simulink subsystem "StateSpaceControllerNominal_SubSystem"  (R2020b)
settings: Solver=VariableStepAuto  StartTime=0.0  StopTime=10.0  RelTol=1e-3
values from neighbouring files (symbols this model uses):
  K = place(A,B,p)    [StateSpaceControllerNominalCont.m]    (also in StateSpaceControllerNominalDigital.m; StateSpaceControllerNominalDirectDigital.m = place(Phi,Gamma,p); StateSpaceControllerRobustCont.m; StateSpaceControllerRobustDigital.m)
  Nu = reshape(Nu,[],1)    [StateSpaceControllerNominalCont.m]    (also in StateSpaceControllerNominalDigital.m; StateSpaceControllerNominalDirectDigital.m; StateSpaceControllerRobustCont.m; StateSpaceControllerRobustDigital.m)
  Nx = reshape(Nx,[],1)    [StateSpaceControllerNominalCont.m]    (also in StateSpaceControllerNominalDigital.m; StateSpaceControllerNominalDirectDigital.m; StateSpaceControllerRobustCont.m; StateSpaceControllerRobustDigital.m)
undefined symbols (not defined in the file or in its folder): rpm2rads
settings Model: Creator=umberto  LastModifiedBy=umberto

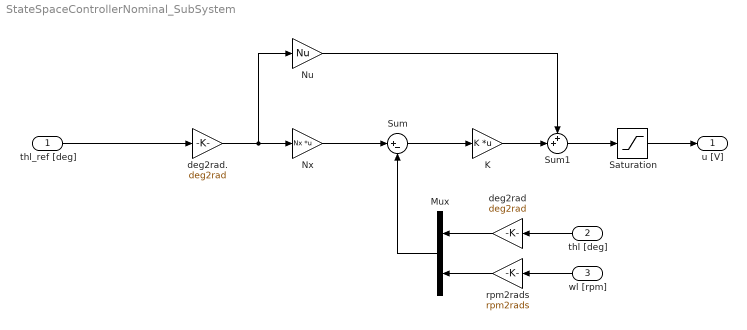
== system StateSpaceControllerNominal_SubSystem ==
  thl_ref [deg] : Inport
  thl [deg] : Inport  Port=2
  wl [rpm] : Inport  Port=3
  K : Gain  Gain=K  Multiplication=Matrix(K*u)
  Mux : Mux  Inputs=2
  Nu : Gain  Gain=Nu
  Nx : Gain  Gain=Nx  Multiplication=Matrix(K*u)
  Saturation : Saturate  UpperLimit=10  LowerLimit=-10
  Sum : Sum  Inputs=|+-
  Sum1 : Sum  Inputs=++|
  deg2rad : Gain  Gain=deg2rad
  deg2rad. : Gain  Gain=deg2rad
  rpm2rads : Gain  Gain=rpm2rads
  u [V] : Outport
  wires:
  deg2rad/1 -> Mux/1
  thl [deg]/1 -> deg2rad/1
  rpm2rads/1 -> Mux/2
  wl [rpm]/1 -> rpm2rads/1
  thl_ref [deg]/1 -> deg2rad./1
  deg2rad./1 -> Nu/1, Nx/1
  Nx/1 -> Sum/1
  Mux/1 -> Sum/2
  Sum/1 -> K/1
  K/1 -> Sum1/2
  Nu/1 -> Sum1/1
  Sum1/1 -> Saturation/1
  Saturation/1 -> u [V]/1
